simulink model "Control_Scheme"  (R2022b)
settings: Solver=VariableStepAuto  StartTime=0.0  StopTime=8.5  RelTol=1e-3
libraries: simulink x1
settings Model: Creator=cster  LastModifiedBy=cster

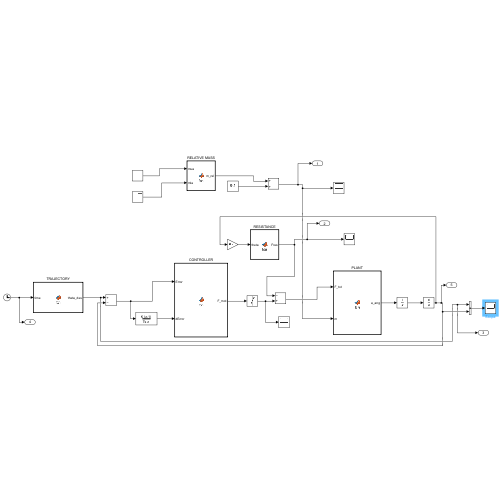
[thumbnail: Simulink's stored preview of the top-level diagram]
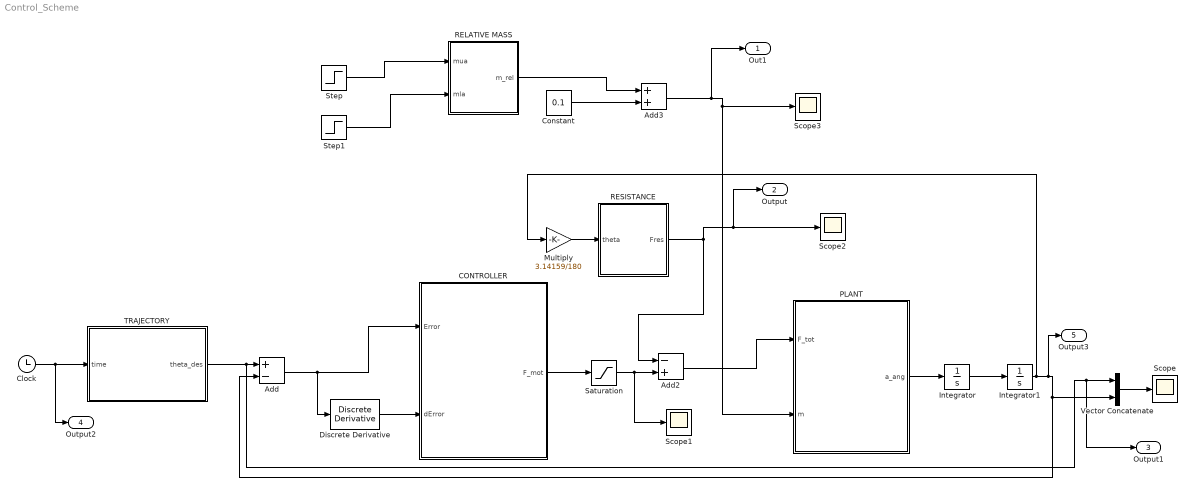
== system Control_Scheme ==
  Add : Sum  Inputs=+-
  Add2 : Sum  Inputs=-+
  Add3 : Sum
  CONTROLLER : MATLAB Function  TreatAsAtomicUnit=on
  Clock : Clock
  Constant : Constant  Value=0.1
  Discrete Derivative : simulink/Discrete/Discrete Derivative  gainval=1.0  ICPrevScaledInput=0.0  OutMin=[]  OutMax=[]  OutDataType=fixdt(1, 16)  OutScaling=2^-10  DoSatur=off
  Integrator : Integrator
  Integrator1 : Integrator
  Multiply : Gain  Gain=3.14159/180
  PLANT : MATLAB Function  TreatAsAtomicUnit=on
  RELATIVE MASS : MATLAB Function  TreatAsAtomicUnit=on
  RESISTANCE : MATLAB Function  TreatAsAtomicUnit=on
  Saturation : Saturate  UpperLimit=0.686/0.015  LowerLimit=-0.686/0.015
  Scope{,1..3} (4 alike) : Scope
  Step : Step  Time=4.5  After=0.03*64.5  SampleTime=0
  Step1 : Step  Time=4.5  After=0.0172*64.5  SampleTime=0
  TRAJECTORY : MATLAB Function  TreatAsAtomicUnit=on
  Vector Concatenate : Concatenate
  Out1 : Outport
  Output : Outport  Port=2
  Output1 : Outport  Port=3
  Output2 : Outport  Port=4
  Output3 : Outport  Port=5
  wires:
  CONTROLLER/1(F_mot) -> Saturation/1
  RESISTANCE/1(Fres) -> Add2/1, Output/1, Scope2/1
  PLANT/1(a_ang) -> Integrator/1
  Integrator/1 -> Integrator1/1
  Add2/1 -> PLANT/1(F_tot)
  Add3/1 -> Out1/1, Scope3/1, PLANT/2(m)
  Constant/1 -> Add3/2
  Step/1 -> RELATIVE MASS/1(mua)
  Integrator1/1 -> Multiply/1, Output3/1, Add/2, Vector Concatenate/2
  Discrete Derivative/1 -> CONTROLLER/2(dError)
  Add/1 -> Discrete Derivative/1, CONTROLLER/1(Error)
  TRAJECTORY/1(theta_des) -> Output1/1, Vector Concatenate/1, Add/1
  Clock/1 -> Output2/1, TRAJECTORY/1(time)
  Vector Concatenate/1 -> Scope/1
  Multiply/1 -> RESISTANCE/1(theta)
  Saturation/1 -> Scope1/1, Add2/2
  Step1/1 -> RELATIVE MASS/2(mla)
  RELATIVE MASS/1(m_rel) -> Add3/1

== matlab function Control_Scheme/PLANT ==
  data: F_tot input; m input; a_ang output
function  a_ang =  fcn(F_tot, m)
%% Knee Controller
% The amount of desired torque should be determinded by knowing the amount
% of desired and actual trajectory of knee.
a = F_tot/m;
a_ang = a/0.3; % a/radius

== matlab function Control_Scheme/CONTROLLER ==
  data: Error input; dError input; F_mot output
function F_mot  = fcn(Error,dError)
%% Controller

kp = 100000;
kd = 5000;

out = kp*Error + kd*dError;

F_mot= out;

== matlab function Control_Scheme/RESISTANCE ==
  data: theta input; Fres output
function  Fres =  fcn(theta)

% Constant gravity of the carriage
m = 0.01;
Fg = sin(theta)*m*9.81;

% Resistance based on the shoulder torque
if theta<(0.5*pi)
    Fres = Fg;
else 
    Length = 0.266+0.2475;
    Weight = 40*9.81;
    shoulder_torque_vec = [0 0.009 0.013 0.017 0.019 0.015 0.0145 0.008 0.005 0]*Length*Weight; % Function taken from reference in article
    angle = linspace(0,180,10);
    shoulder_torque =  interp1(angle,shoulder_torque_vec, rad2deg(theta));
    r = 0.3; %Radius in meters

    Fshoulder = shoulder_torque/r;
    Fres = Fg+Fshoulder;
end

== matlab function Control_Scheme/TRAJECTORY ==
  data: theta_des output; time input
function theta_des = fcn(time)
    theta_des = 20*time; 
end

== matlab function Control_Scheme/RELATIVE MASS ==
  data: mua input; m_rel output; mla input
function  m_rel =  fcn(mua, mla)

Lua = 0.2848; % Length upper arm
Lla = 0.2665; % Length lower arm
r = 0.3; % radius circle arc


rel_dis_UA = 0.5*Lua/r; % ratio between center of mass (UA) distance from shoulder and carriage distance from shoulder.
rel_dis_LA = (0.5*Lla+Lua)/r; % ratio between center of mass (LA) distance from shoulder and carriage distance from shoulder.

m_rel = mua*rel_dis_UA + mla*rel_dis_LA; % relative mass pushed away at the carriage
